simulink model "Flapping_Plant"  (R2017a)
settings: Solver=ode4  StartTime=0.0  StopTime=Tf  FixedStep=0.01  RelTol=1e-3
values from neighbouring files (symbols this model uses):
  A = 0.1    [Energy.m]    (also in Initialize_D2.m = 20)
  a0 = pi/4    (= 0.785398163397)    [Energy.m]    (also in Initialize_D2.m)
  Alpha0 = pi/6    (= 0.523598775598)    [Energy.m]    (also in Initialize_D2.m)
  Alpha_dot0 = 0    [Energy.m]    (also in Initialize_D2.m)
  k = 20    [Energy.m]    (also in Initialize_D2.m = 32)
  Theta0 = 0    [Energy.m]    (also in Initialize_D2.m = 1.0471975512)
  Theta_dot0 = 0    [Energy.m]    (also in Initialize_D2.m)
  w = 4    [Energy.m]    (also in Initialize_D2.m = 120)
  zigma = 10    [Energy.m]    (also in Initialize_D2.m = 0.9)
libraries: dspsrcs4 x1
settings Model: Creator=Amir  LastModifiedBy=Amir
settings SFSimCC: SimUseLocalCustomCode=on
settings RTWCC: RTWUseLocalCustomCode=on

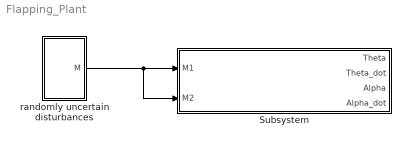
== system Flapping_Plant ==
  Subsystem : Subsystem
  randomly uncertain disturbances : Subsystem
  wires:
  randomly uncertain disturbances/1(M) -> Subsystem/2(M2), Subsystem/1(M1)

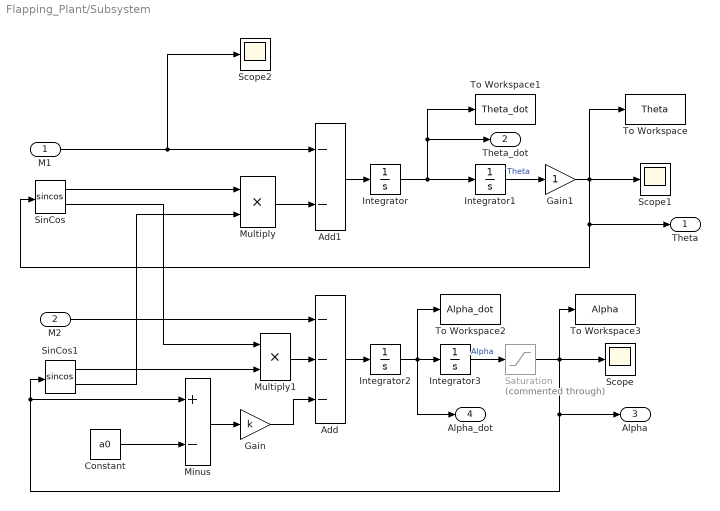
== system Flapping_Plant/Subsystem ==
  M1 : Inport
  M2 : Inport  Port=2
  Add : Sum  Inputs=---
  Add1 : Sum  Inputs=--
  Constant : Constant  Value=a0
  Gain : Gain  Gain=k
  Gain1 : Gain
  Integrator : Integrator  InitialCondition=Theta_dot0
  Integrator1 : Integrator  InitialCondition=Theta0
  Integrator2 : Integrator  InitialCondition=Alpha_dot0
  Integrator3 : Integrator  InitialCondition=Alpha0
  Minus : Sum  Inputs=+-
  Multiply : Product
  Multiply1 : Product
  Saturation : Saturate  Commented=through  UpperLimit=inf  LowerLimit=a0
  Scope : Scope
  Scope1 : Scope
  Scope2 : Scope
  SinCos : Trigonometry  Operator=sincos
  SinCos1 : Trigonometry  Operator=sincos
  To Workspace : ToWorkspace  VariableName=Theta  SampleTime=-1
      settings: Save2DSignal=2-D array (concatenate along first dimension)
  To Workspace1 : ToWorkspace  VariableName=Theta_dot  SampleTime=-1
      settings: Save2DSignal=2-D array (concatenate along first dimension)
  To Workspace2 : ToWorkspace  VariableName=Alpha_dot  SampleTime=-1
      settings: Save2DSignal=2-D array (concatenate along first dimension)
  To Workspace3 : ToWorkspace  VariableName=Alpha  SampleTime=-1
      settings: Save2DSignal=2-D array (concatenate along first dimension)
  Theta : Outport
  Theta_dot : Outport  Port=2
  Alpha : Outport  Port=3
  Alpha_dot : Outport  Port=4
  wires:
  Minus/1 -> Gain/1
  Integrator1/1 -> Gain1/1  "Theta"
  Integrator/1 -> Theta_dot/1, To Workspace1/1, Integrator1/1
  Saturation/1 -> To Workspace3/1, Alpha/1, Minus/1, SinCos1/1, Scope/1
  M1/1 -> Scope2/1, Add1/1
  Integrator2/1 -> Alpha_dot/1, To Workspace2/1, Integrator3/1
  SinCos/2 -> Multiply1/1
  SinCos1/1 -> Multiply1/2
  Multiply1/1 -> Add/2
  Gain/1 -> Add/3
  Integrator3/1 -> Saturation/1  "Alpha"
  Add1/1 -> Integrator/1
  Multiply/1 -> Add1/2
  M2/1 -> Add/1
  SinCos1/2 -> Multiply/2
  Constant/1 -> Minus/2
  Add/1 -> Integrator2/1
  SinCos/1 -> Multiply/1
  Gain1/1 -> Theta/1, SinCos/1, To Workspace/1, Scope1/1

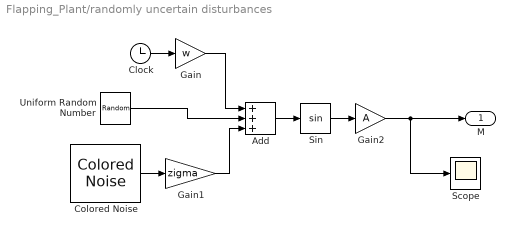
== system Flapping_Plant/randomly uncertain disturbances ==
  Add : Sum  Inputs=+++
  Clock : Clock
  Colored Noise : dspsrcs4/Colored Noise  Color=brown  InverseFrequencyPower=1  NumChannels=1  OutputDataType=double  SamplesPerFrame=1  SampleTime=1  RandomStream=mt19937ar with seed  Seed=67  SimulateUsing=Interpreted execution
      settings: SourceProductName=DSP System Toolbox  SourceProductBaseCode=DS
  Gain : Gain  Gain=w
  Gain1 : Gain  Gain=zigma
  Gain2 : Gain  Gain=A
  Scope : Scope
  Sin : Trigonometry
  Uniform Random Number : UniformRandomNumber  Minimum=0  Maximum=2*pi  SampleTime=1
  M : Outport
  wires:
  Clock/1 -> Gain/1
  Colored Noise/1 -> Gain1/1
  Gain1/1 -> Add/3
  Uniform Random Number/1 -> Add/2
  Gain/1 -> Add/1
  Add/1 -> Sin/1
  Sin/1 -> Gain2/1
  Gain2/1 -> Scope/1, M/1
